simulink model "pendulum_3a113"  (R2018b)
settings: Solver=VariableStepAuto  StartTime=0.0  StopTime=500  RelTol=1e-3
values from neighbouring files (symbols this model uses):
  A = [0 0 1 0;0 0 0 1;0 -Rod_m*g/Cart_m -(Kg^2)*Km*Kb/(Cart_m*Rm*motor_radius^2) 0 ... (first row only)    [pendulum_version1.m]
  B = [0;0;Km*Kg/(Cart_m*Rm*motor_radius);-Km*Kg/(Cart_m*Rm*motor_radius*Rod_l)]    [pendulum_version1.m]
  C = [1 0 0 0 ... (first row only)    [pendulum_version1.m]
  D = [0 ... (first row only)    [pendulum_version1.m]
  K = lqr(A,B,Q,R)    [pendulum_version1.m]
  Ts = 1/200    (= 0.005)    [pendulum_version1.m]
undefined symbols (not defined in the file or in its folder): omega_c
libraries: simulink x1, simulink_extras x1
settings Model: Creator=paul-emileverleye  LastModifiedBy=Kyle
settings DebuggingCC: LibraryContextMissingDiagnostic=none
settings SFSimCC: SimUseLocalCustomCode=off
settings RTWCC: RTWUseLocalCustomCode=off

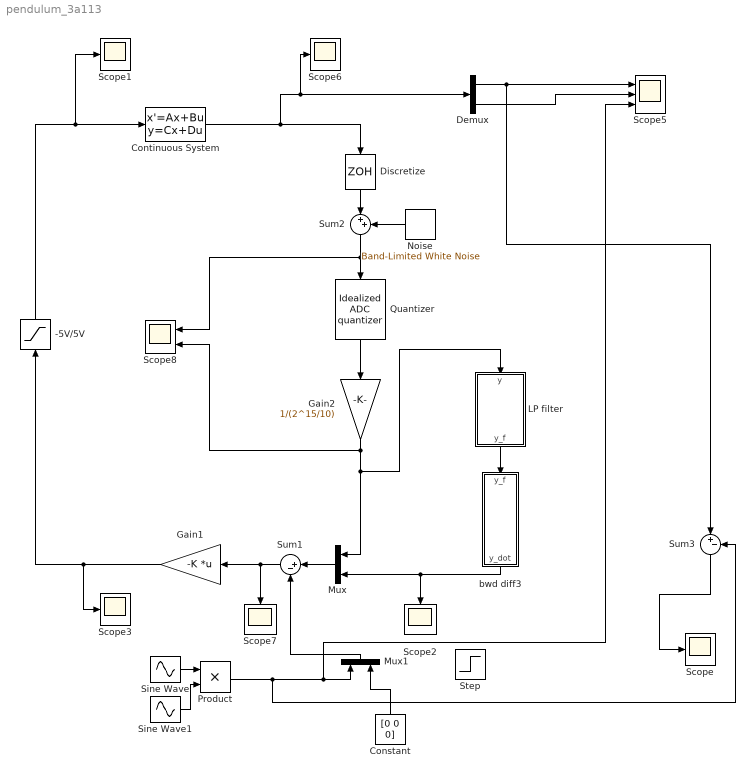
== system pendulum_3a113 ==
  -5V/5V : Saturate  UpperLimit=5  LowerLimit=-5
  Constant : Constant  Value=[0 0 0]
  Continuous System : StateSpace  A=A  B=B  C=C  D=D  InitialCondition=0
  Demux : Demux  Outputs=2
  Discretize : ZeroOrderHold  SampleTime=1/200
  Gain1 : Gain  Gain=-K  Multiplication=Matrix(K*u)
  Gain2 : Gain  Gain=1/(2^15/10)
  LP filter : Subsystem
  Mux : Mux  Inputs=2
  Mux1 : Mux  Inputs=2
  Noise : simulink/Sources/Band-Limited White Noise  Cov=[5e-6; 5e-6]  Ts=1/200  seed=[23341]
  Product : Product
  Quantizer : simulink_extras/Additional Discrete/Idealized ADC quantizer  NumberOfConverterBits=16  Vmin=-10  Vmax=10  OutputDataType=double  OutputNegativeValues=on
      settings: SourceProductName=Simulink
  Scope{,1..3,6..7} (6 alike) : Scope
  Scope5 : Scope  NumInputPorts=3
  Scope8 : Scope  NumInputPorts=2
  Sine Wave : Sin  Frequency=0.1  SampleTime=0
  Sine Wave1 : Sin  Frequency=0.01  SampleTime=0
  Step : Step  After=[1 0 0 0]  SampleTime=0
  Sum1 : Sum  Inputs=|+-
  Sum2 : Sum  Inputs=|++
  Sum3 : Sum  Inputs=|+-
  bwd diff3 : Subsystem
  wires:
  -5V/5V/1 -> Continuous System/1, Scope1/1
  Demux/1 -> Sum3/1, Scope5/1
  Continuous System/1 -> Demux/1, Scope6/1, Discretize/1
  Demux/2 -> Scope5/2
  Sum1/1 -> Scope7/1, Gain1/1
  Noise/1 -> Sum2/2
  Discretize/1 -> Sum2/1
  Sum2/1 -> Scope8/1, Quantizer/1
  Mux/1 -> Sum1/1
  Quantizer/1 -> Gain2/1
  Gain2/1 -> Scope8/2, LP filter/1(y), Mux/1
  Sine Wave/1 -> Product/1
  Sine Wave1/1 -> Product/2
  bwd diff3/1(y_dot) -> Scope2/1, Mux/2
  LP filter/1(y_f) -> bwd diff3/1(y_f)
  Gain1/1 -> Scope3/1, -5V/5V/1
  Mux1/1 -> Sum1/2
  Product/1 -> Sum3/2, Scope5/3, Mux1/1
  Constant/1 -> Mux1/2
  Sum3/1 -> Scope/1

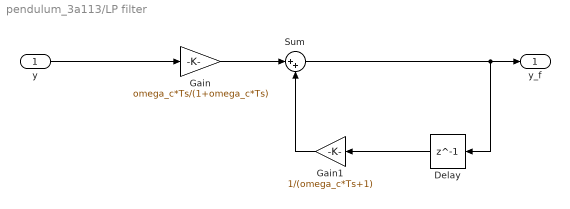
== system pendulum_3a113/LP filter ==
  y : Inport
  Delay : Delay  DelayLength=1  InitialCondition=0
  Gain : Gain  Gain=omega_c*Ts/(1+omega_c*Ts)
  Gain1 : Gain  Gain=1/(omega_c*Ts+1)
  Sum : Sum  Inputs=|++
  y_f : Outport
  wires:
  y/1 -> Gain/1
  Gain/1 -> Sum/1
  Delay/1 -> Gain1/1
  Gain1/1 -> Sum/2
  Sum/1 -> Delay/1, y_f/1

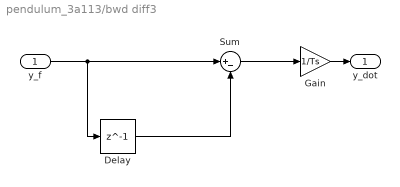
== system pendulum_3a113/bwd diff3 ==
  y_f : Inport
  Delay : Delay  DelayLength=1  InitialCondition=0
  Gain : Gain  Gain=1/Ts
  Sum : Sum  Inputs=|+-
  y_dot : Outport
  wires:
  y_f/1 -> Sum/1, Delay/1
  Gain/1 -> y_dot/1
  Delay/1 -> Sum/2
  Sum/1 -> Gain/1
